simulink model "Tesla_Model_S_P85"  (R2022b)
settings: Solver=VariableStepAuto  StartTime=0.0  StopTime=30  RelTol=1e-3
InitFcn:
  | r = 0.24; % wheel_raduis(meters)
  | Gr = 9.73; % gear ratio
  | m_t_c = 0.25; % Motor Torque Constant
  | b_emf_c = 0.12; % Back EMF Constant
  | l = 493*10^-9; % Inductance of the motor
  | R = 5.3*10^-3; % Armacture Resistance
  | max_T = 601; % max torque of the motor(Nm)
libraries: slpidlib x1
settings Model: Creator=vikram  LastModifiedBy=vikram

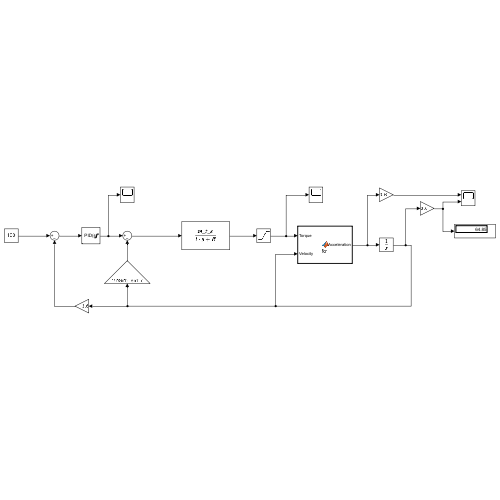
[thumbnail: Simulink's stored preview of the top-level diagram]
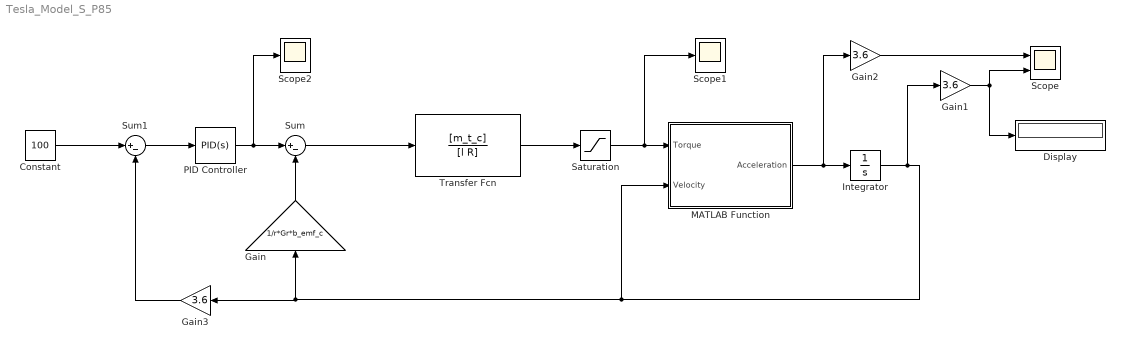
== system Tesla_Model_S_P85 ==
  Constant : Constant  Value=100
  Display : Display
  Gain : Gain  Gain=1/r*Gr*b_emf_c
  Gain1 : Gain  Gain=3.6
  Gain2 : Gain  Gain=3.6
  Gain3 : Gain  Gain=3.6
  Integrator : Integrator
  MATLAB Function : MATLAB Function  TreatAsAtomicUnit=on
  PID Controller : slpidlib/PID Controller  Controller=PID  Form=Parallel  TimeDomain=Continuous-time  UseExternalTs=off  SampleTime=-1  IntegratorMethod=Forward Euler  FilterMethod=Forward Euler  ControllerParametersSource=internal  P=20  I=0.9  UseKiTs=off  D=0.5  N=100  UseFilter=on  TunerSelectOption=Transfer Function Based (PID Tuner App)  InitialConditionSource=internal  InitialConditionForIntegrator=0  InitialConditionForFilter=0  DifferentiatorICPrevScaledInput=0  ExternalReset=none  TrackingMode=off  Kt=1  LimitOutput=on  SatLimitsSource=internal  UpperSaturationLimit=346  LowerSaturationLimit=-346  LinearizeAsGain=on  AntiWindupMode=none  Kb=1  LimitIntegrator=off  UpperIntegratorSaturationLimit=inf  LowerIntegratorSaturationLimit=-inf  POutMin=[]  POutMax=[]  IOutMin=[]  IOutMax=[]  DOutMin=[]  DOutMax=[]  NOutMin=[]  NOutMax=[]  SumOutMin=[]  SumOutMax=[]  SaturationOutMin=[]  SaturationOutMax=[]  PParamMin=[]  PParamMax=[]  IParamMin=[]  IParamMax=[]  DParamMin=[]  DParamMax=[]  NParamMin=[]  NParamMax=[]  KbParamMin=[]  KbParamMax=[]  KtParamMin=[]  KtParamMax=[]  KbOutMin=[]  KbOutMax=[]  KtOutMin=[]  KtOutMax=[]  IntegratorOutMin=[]  IntegratorOutMax=[]  FilterOutMin=[]  FilterOutMax=[]  SumI1OutMin=[]  SumI1OutMax=[]  SumI2OutMin=[]  SumI2OutMax=[]  SumI3OutMin=[]  SumI3OutMax=[]  SumI4OutMin=[]  SumI4OutMax=[]  SumDOutMin=[]  SumDOutMax=[]  DifferentiatorOutMin=[]  DifferentiatorOutMax=[]  FilterDiffOutCoefMin=[]  FilterDiffOutCoefMax=[]  ReciprocalOutMin=[]  ReciprocalOutMax=[]  SumDenOutMin=[]  SumDenOutMax=[]  SumNumOutMin=[]  SumNumOutMax=[]  DivideOutMin=[]  DivideOutMax=[]  UdiffTsProdOutMin=[]  UdiffTsProdOutMax=[]  NTsProdOutMin=[]  NTsProdOutMax=[]  UintegralTsProdOutMin=[]  UintegralTsProdOutMax=[]  UngainTsProdOutMin=[]  UngainTsProdOutMax=[]  ClampingZeroOutDataTypeStr=Inherit: Inherit via back propagation  ClampingZeroOutMin=[]  ClampingZeroOutMax=[]  FilterDenConstantOutDataTypeStr=Inherit: Inherit via back propagation  FilterDenConstantOutMin=[]  FilterDenConstantOutMax=[]  PCopyOutDataTypeStr=Inherit: Inherit via back propagation  PCopyOutMin=[]  PCopyOutMax=[]  NCopyOutDataTypeStr=Inherit: Inherit via back propagation  NCopyOutMin=[]  NCopyOutMax=[]  IntegratorContinuousStateAttributes=''  IntegratorStateMustResolveToSignalObject=off  IntegratorRTWStateStorageClass=Auto  FilterContinuousStateAttributes=''  FilterStateMustResolveToSignalObject=off  FilterRTWStateStorageClass=Auto  ParallelPVariant=InternalParameters  IdealPVariant=Disabled  IVariant=InternalParameters  DVariant=InternalParameters  IntegratorVariant=Continuous  SatVariant=Enabled  AWVariant=Passthrough  PCopyVariant=Disabled  TRVariant=Disabled  FdbkBlocksVariant=Forward  IdealPFdbkVariant=Disabled  SatFdbkVariant=Disabled  DerivativeFilterVariant=ContFilter  NVariant=InternalParameters  NCopyVariant=Disabled  FilterICVariant=InternalICsFilter  IntegratorICVariant=InternalICs  ExternalResetVariant=Disabled  TRSumVariant=Passthrough  SumFdbkVariant=Disabled  SumVariant=Sum_PID  TsampFilterVariant=InternalTs  TsampNgainVariant=Passthrough  TsampIntegralVariant=Passthrough  ExternalSaturationOutDataTypeStr=Inherit: Same as second input
  Saturation : Saturate  UpperLimit=max_T  LowerLimit=-max_T
  Scope : Scope  NumInputPorts=2
  Scope1 : Scope
  Scope2 : Scope
  Sum : Sum  Inputs=|+-
  Sum1 : Sum  Inputs=|+-
  Transfer Fcn : TransferFcn  Numerator=[m_t_c]  Denominator=[l R]
  wires:
  Gain/1 -> Sum/2
  Transfer Fcn/1 -> Saturation/1
  MATLAB Function/1(Acceleration) -> Gain2/1, Integrator/1
  Integrator/1 -> Gain1/1, MATLAB Function/2(Velocity), Gain/1, Gain3/1
  Gain1/1 -> Display/1, Scope/2
  Gain2/1 -> Scope/1
  Sum/1 -> Transfer Fcn/1
  Saturation/1 -> Scope1/1, MATLAB Function/1(Torque)
  PID Controller/1 -> Scope2/1, Sum/1
  Sum1/1 -> PID Controller/1
  Constant/1 -> Sum1/1
  Gain3/1 -> Sum1/2

== matlab function Tesla_Model_S_P85/MATLAB Function ==
  data: Torque input; Acceleration output; Velocity input
function Acceleration = fcn(Torque,Velocity)
r = 0.24; % wheel_radius(meters)
Gr = 9.73; % gear ratio
rho = 1.225; % air density(kg/m^3)
S = 2.3; % frontal area(m^2)
Cd = 0.24; % Coefficient of Drag
Cr = 0.02; % rolling resistance Coefficient
m = 2108; % Mass of the car(kg)
g = 9.81; % gravitational constant
ef = 0.6; % overall efficiency

Acceleration = ((Torque/r*Gr)*ef-(0.5*rho*Velocity^2* S*Cd)-(Cr*m*g))/m;
